simulink subsystem "LC_Battery"  (R2022a)
settings: Solver=VariableStepAuto  StartTime=0.0  StopTime=10.0  RelTol=1e-3
values from neighbouring files (symbols this model uses):
  AN = sim.AN    [getLCParam.m]    (also in runSimulink.m = sim_in.AN)
  C_plant = Slink.C_plant    [runSimulink.m]
  CA = sim.CA    [getLCParam.m]    (also in runSimulink.m = sim_in.CA)
  CONS = sim.CONS    [getLCParam.m]    (also in runSimulink.m = sim_in.CONS)
  EL = sim.EL    [getLCParam.m]    (also in runSimulink.m = sim_in.EL)
  FLAG = sim.FLAG    [getLCParam.m]    (also in runSimulink.m = sim_in.FLAG)
  K_plant = LC_param.K    [runSimulink.m]
  M_cross = V*S_cross*U'    [getLCParam.m]    (also in runSimulink.m = LC_param.M_cross)
  N = sim.N    [getLCParam.m]    (also in runSimulink.m = sim_in.N)
  P = obsv_r(1:end-N_outputs,:)    [HoKalmanReduction.m]    (also in getLCParam.m = sim.P; runSimulink.m = sim_in.P)
  PROPS = sim.PROPS    [getLCParam.m]    (also in runSimulink.m = sim_in.PROPS)
  SEP = sim.SEP    [getLCParam.m]    (also in runSimulink.m = sim_in.SEP)
  SIM = sim.SIM    [getLCParam.m]    (also in runSimulink.m = rmfield(SIM,'Controller_MO_File'))
  SV_IC = SIM.SV_IC    [getLCParam.m]    (also in runSimulink.m = sim_in.SIM.SV_IC)
  U_NV_NT = U_null*V_null'    [getLCParam.m]    (also in runSimulink.m = LC_param.U_NV_NT)
settings Model: Creator=tyevans  LastModifiedBy=tyevans

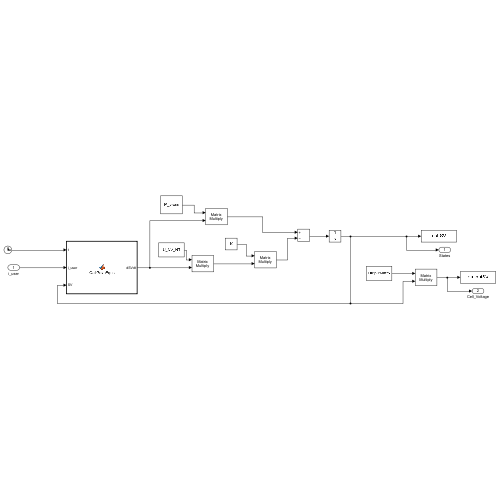
[thumbnail: Simulink's stored preview of the top-level diagram]
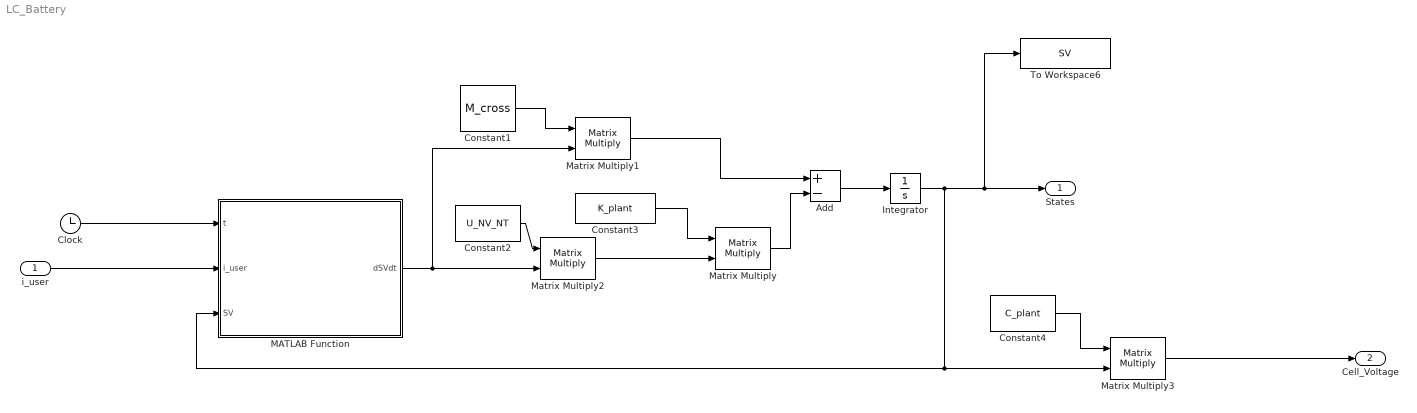
== system LC_Battery ==
  i_user : Inport
  Add : Sum  Inputs=+-
  Clock : Clock
  Constant1 : Constant  Value=M_cross  VectorParams1D=off
  Constant2 : Constant  Value=U_NV_NT  VectorParams1D=off
  Constant3 : Constant  Value=K_plant  VectorParams1D=off
  Constant4 : Constant  Value=C_plant  VectorParams1D=off
  Integrator : Integrator  InitialCondition=SV_IC
  MATLAB Function : MATLAB Function  TreatAsAtomicUnit=on
  Matrix Multiply{,1..3} (4 alike) : Product  Multiplication=Matrix(*)
  To Workspace6 : ToWorkspace  VariableName=SV  SaveFormat=Structure With Time  SampleTime=-1
  States : Outport
  Cell_Voltage : Outport  Port=2
  wires:
  Add/1 -> Integrator/1
  Clock/1 -> MATLAB Function/1(t)
  Integrator/1 -> Matrix Multiply3/2, MATLAB Function/3(SV), States/1, To Workspace6/1
  Constant3/1 -> Matrix Multiply/1
  Matrix Multiply1/1 -> Add/1
  Constant2/1 -> Matrix Multiply2/1
  MATLAB Function/1(dSVdt) -> Matrix Multiply2/2, Matrix Multiply1/2
  Constant4/1 -> Matrix Multiply3/1
  Constant1/1 -> Matrix Multiply1/1
  Matrix Multiply/1 -> Add/2
  Matrix Multiply2/1 -> Matrix Multiply/2
  i_user/1 -> MATLAB Function/2(i_user)
  Matrix Multiply3/1 -> Cell_Voltage/1

== matlab function LC_Battery/MATLAB Function ==
  data: t input; i_user input; dSVdt output; SV input; AN parameter; CA parameter; SEP parameter; EL parameter; SIM parameter; CONS parameter; P parameter; N parameter; FLAG parameter; PROPS parameter
function dSVdt = CallGovnEqns(t,i_user,SV, AN, CA, SEP, EL, SIM, CONS, P, N, FLAG, PROPS)
% Initialize Output
dSVdt = zeros(N.N_SV_tot,1);

% Call GovnEqns
coder.extrinsic('ConvertStrCallGov')
[dSVdt] = ConvertStrCallGov(t,SV,AN,CA,SEP,EL,SIM,CONS,P,N,FLAG,PROPS,i_user);

end
